simulink model "Exp_3_batch_17_Simulation (3)"  (R2020a)
settings: Solver=VariableStepAuto  StartTime=0.0  StopTime=20  RelTol=1e-3
settings Model: Creator=sundaram bhupathi  LastModifiedBy=tarun

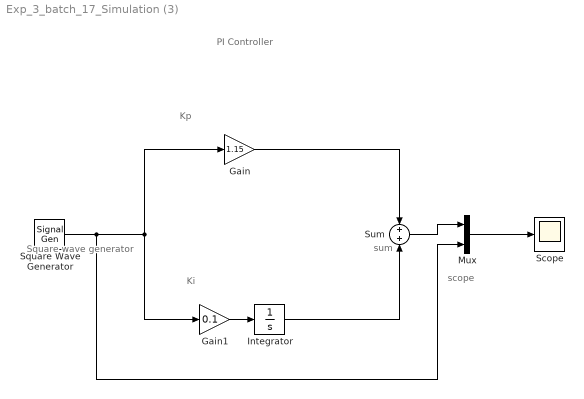
== system Exp_3_batch_17_Simulation (3) ==
  note: Ki
  note: Kp
  note: PI Controller
  note: scope
  note: Square wave generator
  note: sum
  Gain : Gain  Gain=1.15
  Gain1 : Gain  Gain=0.1
  Integrator : Integrator
  Mux : Mux  Inputs=2
  Scope : Scope
  Square Wave Generator : SignalGenerator  WaveForm=square  Amplitude=10  Units=rad/sec
  Sum : Sum  InputSameDT=on  SaturateOnIntegerOverflow=on  OutDataTypeStr=Inherit: Same as first input
  wires:
  Gain/1 -> Sum/1
  Integrator/1 -> Sum/2
  Sum/1 -> Mux/1
  Mux/1 -> Scope/1
  Gain1/1 -> Integrator/1
  Square Wave Generator/1 -> Gain/1, Gain1/1, Mux/2
